simulink model "Excavator_Param_BOFTOF_Calc"  (R2026a)
settings: Solver=ode45  AbsTol=1e-3  EnableMultiTasking=on
PostLoadFcn:
  | if(~exist('bucketForceAngleBOF','var'))
  |    disp('Defining default force angles');
  |    bucketForceAngleBOF = -11.7417;
  |    bucketForceAngleTOF= -1.4472;
  |    bucketForceAngleGravity = -55.5751;
  | end
undefined symbols (not defined in the file or in its folder): A1, A2, B1, B2, B3, BOFTOF_BoomCylArea, BOFTOF_BucketCylArea, BOFTOF_StickCylArea, C1, C2, C3, C4, D1, D2, excv_data, forceTestMaxActiveCylPr, forceTestMaxReactiveCylPr, X, Y, Z
libraries: Excavator_Parts_Param_Lib x21, nesl_utility x12, sm_lib x11, simulink x3, Arrowhead_Lib x1, fl_lib x1
Description:
  | Copyright 2022-2026 The MathWorks, Inc.
settings Model: Creator=smiller  LastModifiedBy=smiller
settings SimscapeCC: ExplicitSolverDiagnosticOptions=none  SimscapeNominalValues="[{\"value\":\"1\",\"unit\":\"A\"},{\"value\":\"1\",\"unit\":\"bar\"},{\"value\":\"1\",\"unit\":\"cm^2\"},{\"value\":\"1\",\"unit\":\"cm^3/s\"},{\"value\":\"1\",\"unit\":\"kJ/kg\"},{\"value\":\"1\",\"unit\":\"kW\"},{\"value\":\"1\",\"unit\":\"l\"},{\"value\":\"1\",\"unit\":\"N\"},{\"value\":\"1\",\"unit\":\"N*m\"},{\"value\":\"1\",\"unit\":\"V\"}]"  SimscapeLogSimulationStatistics=on
settings ExplorerConfigSet: InternalSimMechanicsExplorerSettings="<ExplorerConfiguration><canonicalview>default</canonicalview><AnimationSetting><BasePlaybackSpeed>1.0</BasePlaybackSpeed><PlaybackSpeedFactor>1.0</PlaybackSpeedFactor></AnimationSetting><TilePanel><TileInfo><Tiles Columns=\"1\" Count=\"1\" Rows=\"1\"><Column Weight=\"1\"/><Row Weight=\"1\"/><Tile Height=\"1\" Width=\"1\" X=\"0\" Y=\"0\"/></Tiles></TileInfo><SceneInfo><SceneViewer><BGColor><R>1</R><G>1</G><B>1</B></BGColor><Camera><DoPerspective>off</DoPerspective><Position><X>6.08519841290746477</X><Y>2.23974465526018696</Y><Z>5.98328318454251473</Z></Position><Center><X>6.08519841290746477</X><Y>2.23974465526018696</Y><Z>1.41634799888379348e-07</Z></Center><Up><X>0</X><Y>1</Y><Z>-0</Z></Up><ViewLimDist>1</ViewLimDist><YLim>4.12210355497723135</YLim><XLim>6.50790764061927973</XLim></Camera></SceneViewer></SceneInfo></TilePanel><MechEditorPanel><Cameras/><GfxPanelCameraMap/><VideoCreator><PlaybackSpeedRatio>1.0</PlaybackSpeedRatio><FrameRate>30</FrameRate><VideoFormat>Motion JPEG AVI</VideoFormat><FrameSize>auto</FrameSize></VideoCreator></MechEditorPanel></ExplorerConfiguration>"

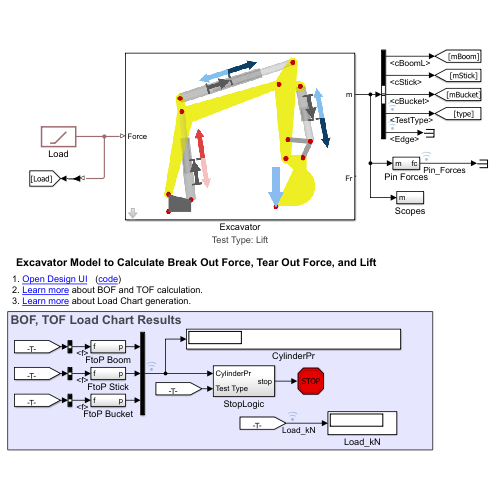
[thumbnail: Simulink's stored preview of the top-level diagram]
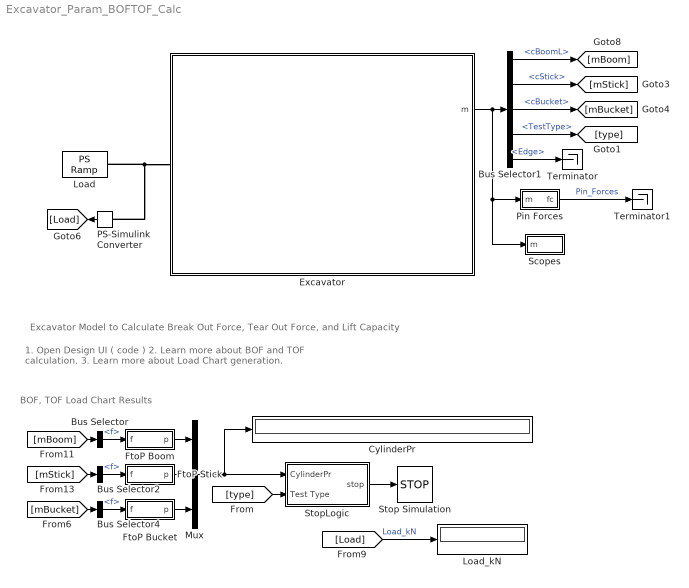
== system Excavator_Param_BOFTOF_Calc ==
  note: BOF, TOF Load Chart Results
  note: Excavator Model to Calculate Break Out Force, Tear Out Force, and Lift Capacity
  note: 1. Open Design UI ( code )
      | 2. Learn more about BOF and TOF calculation.
      | 3. Learn more about Load Chart generation.
  Bus Selector : BusSelector  OutputSignals=f
  Bus Selector1 : BusSelector  OutputSignals=cBoomL,cStick,cBucket,TestType,Edge
  Bus Selector2 : BusSelector  OutputSignals=f
  Bus Selector4 : BusSelector  OutputSignals=f
  CylinderPr : Display
  Excavator : Subsystem  mask{test_type=Lift}
      mask prompts: test_type "Test Type"
      mask init:
      | set_param([gcb '/Apply Force'],'test_type',get_param(gcb,'test_type'));
      | switch(test_type)
      |     case 1
      |         set_param([gcb '/Test Type'],'Value','1');
      |         set_param([gcb '/Mechanism Configuration'],'UniformGravity','None');
      |     case 2
      |         set_param([gcb '/Test Type'],'Value','2');
      |         set_param([gcb '/Mechanism Configuration'],'UniformGravity','None');
      |     case 3
      |         set_param([gcb '/Test Type'],'Value','3');
      |         set_param([gcb '/Mechanism Configuration'],'UniformGravity','Constant');
      | 
      | end
      settings: AttributesFormatString=Test Type: %<test_type>
      mask TypeOptions test_type: BOF | TOF | Lift
      mask Display:
      | switch(get_param(gcb,'test_type'))
      |     case 'BOF'
      |         image('Excavator_Param_Full_CalcForce_BOF_IMAGE.png');
      |     case 'TOF'
      |         image('Excavator_Param_Full_CalcForce_TOF_IMAGE.png');
      |     case 'Lift'
      |         image('Excavator_Param_Full_CalcForce_LoadChart_IMAGE.png');
      | end
  FtoP Boom : Subsystem
  FtoP Bucket : Subsystem
  FtoP Stick : Subsystem
  Load : fl_lib/Physical Signals/Sources/PS Ramp  slope=100 kN/s  start_time=0 s  initial_output=0 kN  ZeroCross=true
  Load_kN : Display
  Mux : Mux  Inputs=3
  PS-Simulink Converter : nesl_utility/PS-Simulink Converter  PhysicalDomain=network_engine_domain  SubClassName=ps_output  LeftPortType=input  RightPortType=output  PseudoPeriodic=off  Frequencies=[]  VectorFormat=inherit  Unit=kN  AffineConversion=off
  Pin Forces : Subsystem
  Scopes : Subsystem
  Stop Simulation : Stop
  StopLogic : Subsystem
  Terminator : Terminator
  Terminator1 : Terminator
  wires:
  PS-Simulink Converter/1 -> [Load]
  Bus Selector1/3 -> [mBucket]  "<cBucket>"
  Excavator/1(m) -> Scopes/1(m), Pin Forces/1(m), Bus Selector1/1
  Bus Selector1/2 -> [mStick]  "<cStick>"
  Bus Selector1/1 -> [mBoom]  "<cBoomL>"
  [mStick] -> Bus Selector2/1
  [mBoom] -> Bus Selector/1
  Bus Selector2/1 -> FtoP Stick/1(f)  "<f>"
  Bus Selector4/1 -> FtoP Bucket/1(f)  "<f>"
  Bus Selector/1 -> FtoP Boom/1(f)  "<f>"
  StopLogic/1(stop) -> Stop Simulation/1
  [Load] -> Load_kN/1  "Load_kN"
  [mBucket] -> Bus Selector4/1
  FtoP Stick/1(p) -> Mux/2
  Mux/1 -> CylinderPr/1, StopLogic/1(CylinderPr)
  FtoP Bucket/1(p) -> Mux/3
  FtoP Boom/1(p) -> Mux/1
  Bus Selector1/4 -> [type]  "<TestType>"
  [type] -> StopLogic/2(Test Type)
  Bus Selector1/5 -> Terminator/1  "<Edge>"
  Pin Forces/1(fc) -> Terminator1/1  "Pin_Forces"
  connections:
  PS-Simulink Converter/LConn1 -- Excavator/LConn1 -- Load/RConn1

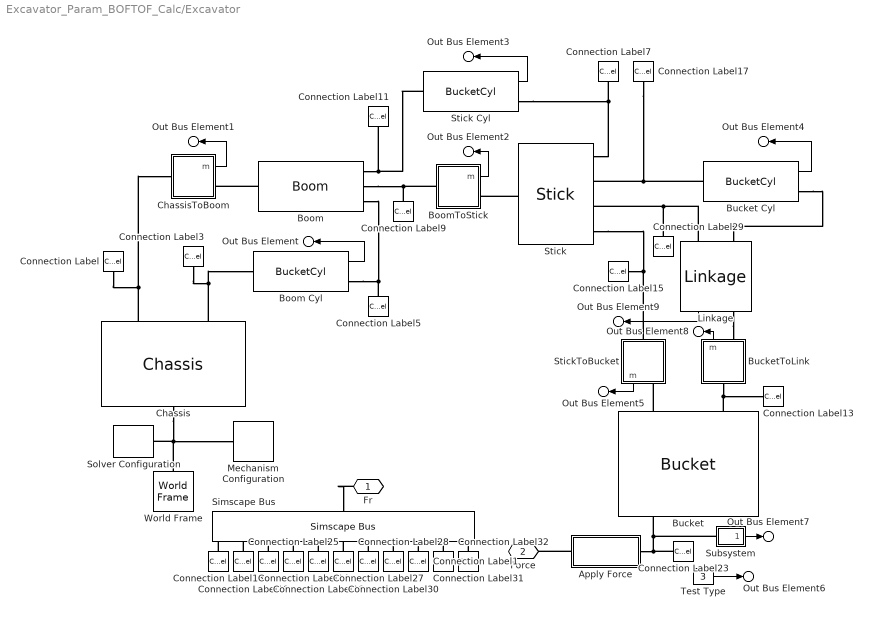
== system Excavator_Param_BOFTOF_Calc/Excavator ==
  Apply Force : Subsystem  mask{test_type=Lift, bof_force_angle=bucketForceAngleBOF, tof_force_angle=bucketForceAngleTOF, lift_force_angle=bucketForceAngleGravity}
      mask prompts: test_type "Test Type"; bof_force_angle "Force Angle, BOF (deg)"; tof_force_angle "Force Angle, TOF (deg)"; lift_force_angle "Force Angle, Lift (deg)"
      mask init:
      | switch(test_type)
      |     case 1
      |         angleCutEdge2BucketForce = bof_force_angle;
      |     case 2
      |         angleCutEdge2BucketForce = tof_force_angle;
      |     case 3
      |         angleCutEdge2BucketForce = lift_force_angle;
      | end
      settings: AttributesFormatString=Test Type: %<test_type>
      mask TypeOptions test_type: BOF | TOF | Lift
  Boom : Excavator_Parts_Param_Lib/Boom  part_thk=excv_data.arm.thk*1.05  part_clr=excv_data.arm.clr  opc=excv_data.arm.opc  pin_len=excv_data.pin.len  pin_rad=excv_data.pin.rad  pin_clr=excv_data.pin.clr  pin_opc=excv_data.pin.opc  Boom=ExcvLocal.Boom  part_mass=LoadChart_BoomMass
  Boom Cyl : Excavator_Parts_Param_Lib/BucketCyl  initPos=initBoomPistonPos  max_force=excv_data.cyl_force.max_force  max_length=excv_data.cyl_force.max_length  arrow_depth=excv_data.cyl_force.depth  line_width=excv_data.cyl_force.line_width  tip_a=90  tip_l=excv_data.cyl_force.tip_length  arrow_clr=excv_data.cyl_force.clr  arrow_opc=excv_data.cyl_force.opc  cyl_len=excv_data.boomcyl.len  cyl_rad=excv_data.cyl.rad  cyl_clr=excv_data.cyl.clr  cyl_opc=excv_data.cyl.opc  pist_len=excv_data.boompist.len  pist_rad=excv_data.pist.rad  pist_clr=excv_data.pist.clr  pist_opc=excv_data.pist.opc
  BoomToStick : Subsystem
      mask Display: image('Excavator_Revolute_IMAGE.png')
  Bucket : Excavator_Parts_Param_Lib/Bucket  part_thk=excv_data.bucket.thk  part_clr=excv_data.bucket.clr  opc=excv_data.arm.opc  pin_len=excv_data.pin.len  pin_rad=excv_data.pin.rad  pin_clr=excv_data.pin.clr  pin_opc=excv_data.pin.opc  Bucket=ExcvLocal.Bucket  part_mass=LoadChart_BucketMass
  Bucket Cyl : Excavator_Parts_Param_Lib/BucketCyl  initPos=initBucketPistonPos  max_force=excv_data.cyl_force.max_force  max_length=excv_data.cyl_force.max_length  arrow_depth=excv_data.cyl_force.depth  line_width=excv_data.cyl_force.line_width  tip_a=90  tip_l=excv_data.cyl_force.tip_length  arrow_clr=excv_data.cyl_force.clr  arrow_opc=excv_data.cyl_force.opc  cyl_len=excv_data.bucketcyl.len  cyl_rad=excv_data.cyl.rad  cyl_clr=excv_data.cyl.clr  cyl_opc=excv_data.cyl.opc  pist_len=excv_data.bucketpist.len  pist_rad=excv_data.pist.rad  pist_clr=excv_data.pist.clr  pist_opc=excv_data.pist.opc
  BucketToLink : Subsystem
      mask Display: image('Excavator_Revolute_IMAGE.png')
  Chassis : Excavator_Parts_Param_Lib/Chassis  Chassis=ExcvLocal.Chassis  opc=excv_data.arm.opc  part_thk=excv_data.chassis.thk  part_clr=excv_data.chassis.clr  pin_clr=excv_data.pin.clr  pin_rad=excv_data.pin.rad  pin_len=excv_data.pin.len  pin_opc=excv_data.pin.opc
  ChassisToBoom : Subsystem
      mask Display: image('Excavator_Revolute_IMAGE.png')
  Connection Label : ConnectionLabel  Label=A1
  Connection Label1 : ConnectionLabel  Label=C4
  Connection Label11 : ConnectionLabel  Label=B2
  Connection Label13 : ConnectionLabel  Label=D1
  Connection Label15 : ConnectionLabel  Label=C4
  Connection Label17 : ConnectionLabel  Label=C2
  Connection Label18 : ConnectionLabel  Label=A1
  Connection Label19 : ConnectionLabel  Label=A2
  Connection Label23 : ConnectionLabel  Label=D2
  Connection Label24 : ConnectionLabel  Label=B1
  Connection Label25 : ConnectionLabel  Label=B2
  Connection Label26 : ConnectionLabel  Label=B3
  Connection Label27 : ConnectionLabel  Label=C1
  Connection Label28 : ConnectionLabel  Label=C2
  Connection Label29 : ConnectionLabel  Label=C3
  Connection Label3 : ConnectionLabel  Label=A2
  Connection Label30 : ConnectionLabel  Label=C3
  Connection Label31 : ConnectionLabel  Label=D1
  Connection Label32 : ConnectionLabel  Label=D2
  Connection Label5 : ConnectionLabel  Label=B1
  Connection Label7 : ConnectionLabel  Label=C1
  Connection Label9 : ConnectionLabel  Label=B3
  Linkage : Excavator_Parts_Param_Lib/Linkage  Linkage=ExcvLocal.Linkage  link_clr=excv_data.link.clr  link_thk=excv_data.link.thk  opc=excv_data.link.opc  pin_clr=excv_data.pin.clr  pin_rad=excv_data.pin.rad  pin_len=excv_data.pin.len  pin_opc=excv_data.pin.opc
  Mechanism Configuration : sm_lib/Utilities/Mechanism Configuration  UniformGravity=Constant  GravityVector=[0 -9.80665 0]  GravityVectorUnits=m/s^2  LinearizationDelta=0.001  JointModeTransitionNonlinearIterations=2
      settings: AttributesFormatString=Gravity: %<UniformGravity>
  Simscape Bus : SimscapeBus  HierarchyStrings=A1;A2;B1;B2;B3;C1;C2;C3;C4;D1;D2
  Solver Configuration : nesl_utility/Solver Configuration  PhysicalDomain=network_engine_domain  SubClassName=solver  LeftPortType=input  RightPortType=generic  Tones=[]  Harmonics=[]  SimulateNoise=off  Profile=off  UseLocalSampling=off  EnableSwitchedLinearOptims=on  FrequencyDomain=off  UseCCode=off  RelTol=0.001  AbsTol=1e-06  MinStep=1e-09  ToWorkspace=off  RevertToSquareIcSolve=off  NumHomotopyIterations=100  PhasorMode=off  PhasorModeNumHarmonics=1  ConsistencySolver=NEWTON_FTOL  CanonicalOrdering=UNORDERED  OptimizeIntermediates=UNOPTIMIZED  IndexReductionMethod=DerivativeReplacement  DoDC=off  ResidualTolerance=1e-09  ConsistencyTolSource=GLOBAL  ConsistencyAbsTol=0.001  ConsistencyRelTol=0.001  ConsistencyTolFactor=0.001  UseLocalSolver=off  LocalSolverChoice=NE_BACKWARD_EULER_ADVANCER  ResolveIndetEquations=on  FunctionEvalNumThread=1  LocalSolverSampleTime=0.001  DoFixedCost=off  MaxNonlinIter=3  MaxModeIter=2  ComputeImpulses=off  ImpulseIterations=2  LinearAlgebra=Sparse  LinearAlgebraNumThread=0  EquationFormulation=NE_TIME_EF  DelaysMemoryBudget=1024  AutomaticFiltering=on  FilteringTimeConstant=0.001  PartitionStorageMethod=AS_NEEDED  PartitionMemoryBudget=1024  PartitionMethod=FAST  MultibodyUseLocalSolver=off  MultibodyLocalSolverChoice=ODE1  MultibodyLocalSolverSampleTime=0.001
  Stick : Excavator_Parts_Param_Lib/Stick  part_thk=excv_data.arm.thk  part_clr=excv_data.arm.clr*0.9  opc=excv_data.arm.opc  pin_len=excv_data.pin.len  pin_rad=excv_data.pin.rad  pin_opc=excv_data.pin.opc  pin_clr=excv_data.pin.clr  Stick=ExcvLocal.Stick  part_mass=LoadChart_StickMass
  Stick Cyl : Excavator_Parts_Param_Lib/BucketCyl  initPos=initStickPistonPos  max_force=excv_data.cyl_force.max_force  max_length=excv_data.cyl_force.max_length  arrow_depth=excv_data.cyl_force.depth  line_width=excv_data.cyl_force.line_width  tip_a=90  tip_l=excv_data.cyl_force.tip_length  arrow_clr=excv_data.cyl_force.clr  arrow_opc=excv_data.cyl_force.opc  cyl_len=excv_data.stickcyl.len  cyl_rad=excv_data.cyl.rad  cyl_clr=excv_data.cyl.clr  cyl_opc=excv_data.cyl.opc  pist_len=excv_data.stickpist.len  pist_rad=excv_data.pist.rad  pist_clr=excv_data.pist.clr  pist_opc=excv_data.pist.opc
  StickToBucket : Subsystem
      mask Display: image('Excavator_Revolute_IMAGE.png')
  Subsystem : Subsystem
  Test Type : Constant  Value=3
  World Frame : sm_lib/Frames and Transforms/World Frame
  Fr : PMIOPort  Side=Right
  Force : PMIOPort  Port=2  Side=Left
  Out Bus Element : Outport  PortName=m  Element=cBoomL
  Out Bus Element3 : Outport  PortName=m  Element=cStick
  Out Bus Element4 : Outport  PortName=m  Element=cBucket
  Out Bus Element1 : Outport  PortName=m  Element=jC2B
  Out Bus Element2 : Outport  PortName=m  Element=jB2S
  Out Bus Element5 : Outport  PortName=m  Element=jS2B
  Out Bus Element6 : Outport  PortName=m  Element=TestType
  Out Bus Element7 : Outport  PortName=m  Element=Edge
  Out Bus Element8 : Outport  PortName=m  Element=jB2L
  Out Bus Element9 : Outport  PortName=m  Element=Linkage
  wires:
  Boom Cyl/1 -> Out Bus Element/1
  Stick Cyl/1 -> Out Bus Element3/1
  Bucket Cyl/1 -> Out Bus Element4/1
  ChassisToBoom/1(m) -> Out Bus Element1/1
  BoomToStick/1(m) -> Out Bus Element2/1
  StickToBucket/1(m) -> Out Bus Element5/1
  Test Type/1 -> Out Bus Element6/1
  Subsystem/1(xy) -> Out Bus Element7/1
  BucketToLink/1(m) -> Out Bus Element8/1
  Linkage/1 -> Out Bus Element9/1
  connections:
  Connection Label24/LConn1 -- Simscape Bus/LConn3
  Connection Label32/LConn1 -- Simscape Bus/LConn11
  Connection Label/LConn1 -- Chassis/RConn1 -- ChassisToBoom/LConn1
  Connection Label29/LConn1 -- Linkage/LConn1 -- Stick/RConn3
  Stick/RConn1 -- Stick Cyl/RConn1 -- Connection Label7/LConn1
  Boom/RConn1 -- Stick Cyl/LConn1 -- Connection Label11/LConn1
  Bucket/LConn1 -- StickToBucket/RConn1
  Connection Label18/LConn1 -- Simscape Bus/LConn1
  Connection Label1/LConn1 -- Simscape Bus/LConn9
  Connection Label5/LConn1 -- Boom Cyl/RConn1 -- Boom/RConn3
  World Frame/RConn1 -- Chassis/LConn1 -- Mechanism Configuration/RConn1 -- Solver Configuration/RConn1
  Connection Label31/LConn1 -- Simscape Bus/LConn10
  Bucket/LConn2 -- Connection Label13/LConn1 -- BucketToLink/LConn1
  Connection Label26/LConn1 -- Simscape Bus/LConn5
  Connection Label28/LConn1 -- Simscape Bus/LConn7
  Connection Label19/LConn1 -- Simscape Bus/LConn2
  Connection Label27/LConn1 -- Simscape Bus/LConn6
  Connection Label25/LConn1 -- Simscape Bus/LConn4
  Connection Label30/LConn1 -- Simscape Bus/LConn8
  Connection Label17/LConn1 -- Bucket Cyl/LConn1 -- Stick/RConn2
  Fr/RConn1 -- Simscape Bus/RConn1
  Connection Label3/LConn1 -- Boom Cyl/LConn1 -- Chassis/RConn2
  Boom/LConn1 -- ChassisToBoom/RConn1
  Connection Label9/LConn1 -- BoomToStick/LConn1 -- Boom/RConn2
  Stick/LConn1 -- BoomToStick/RConn1
  StickToBucket/LConn1 -- Connection Label15/LConn1 -- Stick/RConn4
  Apply Force/LConn1 -- Force/RConn1
  Apply Force/RConn1 -- Connection Label23/LConn1 -- Bucket/RConn1 -- Subsystem/LConn1
  Bucket Cyl/RConn1 -- Linkage/LConn2
  Linkage/RConn1 -- BucketToLink/RConn1

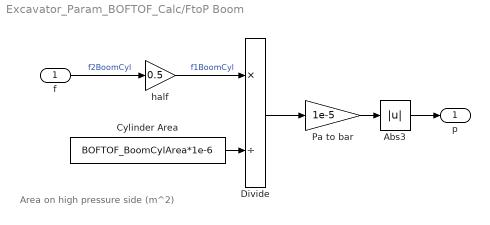
== system Excavator_Param_BOFTOF_Calc/FtoP Boom ==
  note: Area on high pressure side (m^2)
  f : Inport
  Abs3 : Abs  SaturateOnIntegerOverflow=off
  Cylinder Area : Constant  Value=BOFTOF_BoomCylArea*1e-6
  Divide : Product  Inputs=*/
  Pa to bar : Gain  Gain=1e-5
  half : Gain  Gain=0.5
  p : Outport
  wires:
  f/1 -> half/1  "f2BoomCyl"
  Divide/1 -> Pa to bar/1
  half/1 -> Divide/1  "f1BoomCyl"
  Abs3/1 -> p/1
  Pa to bar/1 -> Abs3/1
  Cylinder Area/1 -> Divide/2

== system Excavator_Param_BOFTOF_Calc/FtoP Bucket ==
  note: Area on high pressure side (m^2)
  f : Inport
  Abs1 : Abs  SaturateOnIntegerOverflow=off
  Cylinder Area : Constant  Value=BOFTOF_BucketCylArea*1e-6
  Divide : Product  Inputs=*/
  Pa to bar : Gain  Gain=1e-5
  p : Outport
  wires:
  f/1 -> Divide/1
  Pa to bar/1 -> Abs1/1
  Divide/1 -> Pa to bar/1
  Abs1/1 -> p/1
  Cylinder Area/1 -> Divide/2

== system Excavator_Param_BOFTOF_Calc/FtoP Stick ==
  note: Area on high pressure side (m^2)
  f : Inport
  Abs3 : Abs  SaturateOnIntegerOverflow=off
  Cylinder Area : Constant  Value=BOFTOF_StickCylArea*1e-6
  Divide : Product  Inputs=*/
  Pa to Bar : Gain  Gain=1e-5
  p : Outport
  wires:
  Abs3/1 -> p/1
  Divide/1 -> Pa to Bar/1
  Pa to Bar/1 -> Abs3/1
  f/1 -> Divide/1
  Cylinder Area/1 -> Divide/2

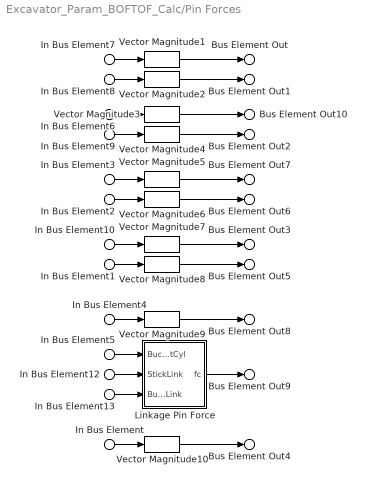
== system Excavator_Param_BOFTOF_Calc/Pin Forces ==
  In Bus Element10 : Inport  PortName=m  Element=cStick.jB.fc
  In Bus Element1 : Inport  PortName=m  Element=cStick.jF.fc
  In Bus Element7 : Inport  PortName=m  Element=jC2B.fc
  In Bus Element8 : Inport  PortName=m  Element=jB2S.fc
  In Bus Element9 : Inport  PortName=m  Element=jS2B.fc
  In Bus Element : Inport  PortName=m  Element=jB2L.fc
  In Bus Element2 : Inport  PortName=m  Element=cBoomL.jB.fc
  In Bus Element3 : Inport  PortName=m  Element=cBoomL.jF.fc
  In Bus Element4 : Inport  PortName=m  Element=cBucket.jB.fc
  In Bus Element5 : Inport  PortName=m  Element=cBucket.jF.fc
  In Bus Element6 : Inport  PortName=m  Element=Linkage.jS2L.fc
  In Bus Element12 : Inport  PortName=m  Element=Linkage.jSL2BC.fc
  In Bus Element13 : Inport  PortName=m  Element=Linkage.jBL2BC.fc
  Linkage Pin Force : Subsystem
  Vector Magnitude{1..10} (10 alike) : Excavator_Parts_Param_Lib/Vector Magnitude  SystemSampleTime=-1  VariantActivationTime=update diagram  EmptyChoice=off  PassThrough=off  PassThroughVariantControl=(default)  EmptyChoiceVariantControl=(default)  AllowFlexibleInterface=on  Latency=0  AutoFrameSizeCalculation=off
  Bus Element Out : Outport  PortName=fc  Element=Boom_To_Chassis
  Bus Element Out1 : Outport  PortName=fc  Element=Boom_To_Stick
  Bus Element Out2 : Outport  PortName=fc  Element=Stick_To_Bucket
  Bus Element Out3 : Outport  PortName=fc  Element=Stick_Cylinder_To_Boom
  Bus Element Out4 : Outport  PortName=fc  Element=Bucket_To_Linkage
  Bus Element Out5 : Outport  PortName=fc  Element=Stick_Cylinder_To_Stick
  Bus Element Out6 : Outport  PortName=fc  Element=Boom_Cylinder_To_Chassis
  Bus Element Out7 : Outport  PortName=fc  Element=Boom_Cylinder_To_Boom
  Bus Element Out8 : Outport  PortName=fc  Element=Bucket_Cylinder_To_Stick
  Bus Element Out9 : Outport  PortName=fc  Element=Bucket_Cylinder_To_Linkage
  Bus Element Out10 : Outport  PortName=fc  Element=Stick_To_Linkage
  wires:
  Vector Magnitude7/1 -> Bus Element Out3/1
  In Bus Element10/1 -> Vector Magnitude7/1
  Vector Magnitude4/1 -> Bus Element Out2/1
  In Bus Element9/1 -> Vector Magnitude4/1
  Vector Magnitude2/1 -> Bus Element Out1/1
  In Bus Element8/1 -> Vector Magnitude2/1
  Vector Magnitude1/1 -> Bus Element Out/1
  In Bus Element7/1 -> Vector Magnitude1/1
  In Bus Element/1 -> Vector Magnitude10/1
  Vector Magnitude10/1 -> Bus Element Out4/1
  Vector Magnitude8/1 -> Bus Element Out5/1
  In Bus Element1/1 -> Vector Magnitude8/1
  In Bus Element2/1 -> Vector Magnitude6/1
  In Bus Element3/1 -> Vector Magnitude5/1
  Vector Magnitude6/1 -> Bus Element Out6/1
  Vector Magnitude5/1 -> Bus Element Out7/1
  In Bus Element4/1 -> Vector Magnitude9/1
  Vector Magnitude9/1 -> Bus Element Out8/1
  In Bus Element6/1 -> Vector Magnitude3/1
  Vector Magnitude3/1 -> Bus Element Out10/1
  In Bus Element5/1 -> Linkage Pin Force/1(BucketCyl)
  In Bus Element12/1 -> Linkage Pin Force/2(StickLink)
  In Bus Element13/1 -> Linkage Pin Force/3(BucketLink)
  Linkage Pin Force/1(fc) -> Bus Element Out9/1

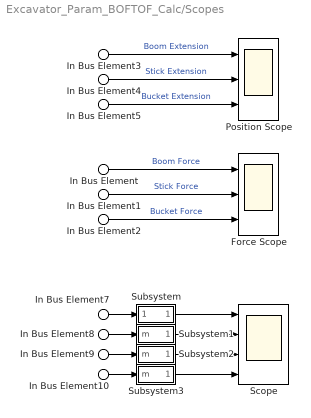
== system Excavator_Param_BOFTOF_Calc/Scopes ==
  In Bus Element : Inport  PortName=m  Element=cBoomL.f
  In Bus Element3 : Inport  PortName=m  Element=cBoomL.pz
  In Bus Element1 : Inport  PortName=m  Element=cStick.f
  In Bus Element4 : Inport  PortName=m  Element=cStick.pz
  In Bus Element10 : Inport  PortName=m  Element=cStick.jB.fc
  In Bus Element2 : Inport  PortName=m  Element=cBucket.f
  In Bus Element5 : Inport  PortName=m  Element=cBucket.pz
  In Bus Element7 : Inport  PortName=m  Element=jC2B.fc
  In Bus Element8 : Inport  PortName=m  Element=jB2S.fc
  In Bus Element9 : Inport  PortName=m  Element=jS2B.fc
  Force Scope : Scope  NumInputPorts=3
      settings: Title=Cylinder Forces  ActiveDisplayYMinimum=-2.01855993393E+6  ActiveDisplayYMaximum=1.89358945982E+6
  Position Scope : Scope  NumInputPorts=3
      settings: ActiveDisplayYMinimum=2036.75361  ActiveDisplayYMaximum=4067.06604
  Scope : Scope  NumInputPorts=4
      settings: ActiveDisplayYMinimum=-225872.14451  ActiveDisplayYMaximum=2.03284930056E+6
  Subsystem : Subsystem
  Subsystem1 : Subsystem
  Subsystem2 : Subsystem
  Subsystem3 : Subsystem
  wires:
  In Bus Element/1 -> Force Scope/1  "Boom Force"
  In Bus Element1/1 -> Force Scope/2  "Stick Force"
  In Bus Element2/1 -> Force Scope/3  "Bucket Force"
  In Bus Element5/1 -> Position Scope/3  "Bucket Extension"
  In Bus Element4/1 -> Position Scope/2  "Stick Extension"
  In Bus Element3/1 -> Position Scope/1  "Boom Extension"
  In Bus Element7/1 -> Subsystem/1(In1)
  Subsystem/1(Out1) -> Scope/1
  In Bus Element8/1 -> Subsystem1/1(m)
  Subsystem1/1(Out1) -> Scope/2
  In Bus Element9/1 -> Subsystem2/1(m)
  Subsystem2/1(Out1) -> Scope/3
  In Bus Element10/1 -> Subsystem3/1(m)
  Subsystem3/1(Out1) -> Scope/4

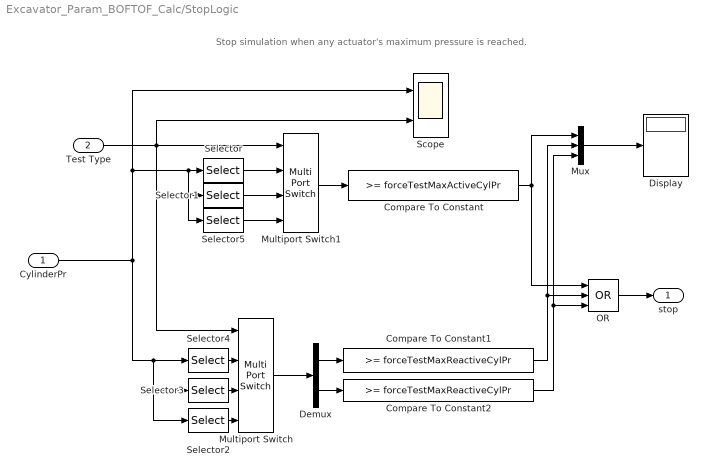
== system Excavator_Param_BOFTOF_Calc/StopLogic ==
  note: Stop simulation when any actuator's maximum pressure is reached.
  CylinderPr : Inport
  Test Type : Inport  Port=2
  Compare To Constant : simulink/Logic and Bit Operations/Compare To Constant  relop=>=  const=forceTestMaxActiveCylPr  OutDataTypeStr=boolean
  Compare To Constant1 : simulink/Logic and Bit Operations/Compare To Constant  relop=>=  const=forceTestMaxReactiveCylPr  OutDataTypeStr=boolean
  Compare To Constant2 : simulink/Logic and Bit Operations/Compare To Constant  relop=>=  const=forceTestMaxReactiveCylPr  OutDataTypeStr=boolean
  Demux : Demux  Outputs=2
  Display : Display
  Multiport Switch : MultiPortSwitch  SaturateOnIntegerOverflow=off  InputSameDT=off
  Multiport Switch1 : MultiPortSwitch  SaturateOnIntegerOverflow=off  InputSameDT=off
  Mux : Mux  Inputs=3
  OR : Logic  Operator=OR  Inputs=3  IconShape=distinctive  AllPortsSameDT=off  OutDataTypeStr=boolean
  Scope : Scope  NumInputPorts=2
      settings: ActiveDisplayYMinimum=-50  ActiveDisplayYMaximum=450
  Selector : Selector  InputPortWidth=3  IndexOptions=Index vector (dialog)  Indices=3  OutputSizes=1
  Selector1 : Selector  InputPortWidth=3  IndexOptions=Index vector (dialog)  Indices=2  OutputSizes=1
  Selector2 : Selector  InputPortWidth=3  IndexOptions=Index vector (dialog)  Indices=[2,3]  OutputSizes=1
  Selector3 : Selector  InputPortWidth=3  IndexOptions=Index vector (dialog)  Indices=[1,3]  OutputSizes=1
  Selector4 : Selector  InputPortWidth=3  IndexOptions=Index vector (dialog)  Indices=[1,2]  OutputSizes=1
  Selector5 : Selector  InputPortWidth=3  IndexOptions=Index vector (dialog)  Indices=1  OutputSizes=1
  stop : Outport
  wires:
  OR/1 -> stop/1
  Compare To Constant2/1 -> OR/3, Mux/3
  Demux/2 -> Compare To Constant2/1
  Demux/1 -> Compare To Constant1/1
  CylinderPr/1 -> Selector4/1, Selector3/1, Selector2/1, Scope/1, Selector5/1, Selector1/1, Selector/1
  Compare To Constant1/1 -> OR/2, Mux/2
  Multiport Switch/1 -> Demux/1
  Compare To Constant/1 -> Mux/1, OR/1
  Multiport Switch1/1 -> Compare To Constant/1
  Selector4/1 -> Multiport Switch/2
  Selector3/1 -> Multiport Switch/3
  Selector1/1 -> Multiport Switch1/3
  Selector/1 -> Multiport Switch1/2
  Mux/1 -> Display/1
  Test Type/1 -> Scope/2, Multiport Switch1/1, Multiport Switch/1
  Selector2/1 -> Multiport Switch/4
  Selector5/1 -> Multiport Switch1/4

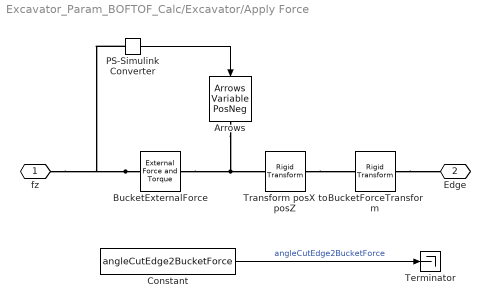
== system Excavator_Param_BOFTOF_Calc/Excavator/Apply Force ==
  Arrows : Arrowhead_Lib/Arrows Variable PosNeg  max_force=4e5  max_length=3  arrow_clr=[0.9019608 0.7058824 0.45490196]  arrow_depth=0.5  line_width=0.2  tip_a=90  tip_l=1  arrow_opc=1
  BucketExternalForce : sm_lib/Forces and Torques/External Force and Torque  EnableForceX=off  EnableForceY=off  EnableForceZ=on  EnableForce=off  ForceResolutionFrame=AttachedFrame  EnableTorqueX=off  EnableTorqueY=off  EnableTorqueZ=off  EnableTorque=off  TorqueResolutionFrame=AttachedFrame
  BucketForceTransform : sm_lib/Frames and Transforms/Rigid Transform  RotationMethod=StandardAxis  FollAlignAxisA=+X  BaseAlignAxisA=+Y  FollAlignAxisB=+Y  BaseAlignAxisB=+Z  RotationStandardAxis=+Z  RotationAngle=angleCutEdge2BucketForce  RotationAngleUnits=deg  RotationArbitraryAxis=[0 0 1]  RotationSequenceAxes=FollowerAxes  RotationSequence=XYX  RotationSequenceAngles=[0 0 0]  RotationSequenceAnglesUnits=deg  RotationMatrix=[1 0 0; 0 1 0; 0 0 1]  Quaternion=[1 0 0 0]  TranslationMethod=None  TranslationCartesianOffset=[0 0 0]  TranslationCartesianOffsetUnits=mm  TranslationStandardAxis=+Z  TranslationStandardOffset=0  TranslationStandardOffsetUnits=mm  TranslationROffset=0  TranslationROffsetUnits=m  TranslationThetaOffset=0  TranslationThetaOffsetUnits=deg  TranslationZOffset=0  TranslationZOffsetUnits=m
  Constant : Constant  Value=angleCutEdge2BucketForce
  PS-Simulink Converter : nesl_utility/PS-Simulink Converter  PhysicalDomain=network_engine_domain  SubClassName=ps_output  LeftPortType=input  RightPortType=output  PseudoPeriodic=off  Frequencies=[]  VectorFormat=inherit  Unit=inherit  AffineConversion=off
  Terminator : Terminator
  Transform posX to posZ : sm_lib/Frames and Transforms/Rigid Transform  RotationMethod=StandardAxis  FollAlignAxisA=+X  BaseAlignAxisA=+Y  FollAlignAxisB=+Y  BaseAlignAxisB=+Z  RotationStandardAxis=+Y  RotationAngle=90  RotationAngleUnits=deg  RotationArbitraryAxis=[0 0 1]  RotationSequenceAxes=FollowerAxes  RotationSequence=XYX  RotationSequenceAngles=[0 0 0]  RotationSequenceAnglesUnits=deg  RotationMatrix=[1 0 0; 0 1 0; 0 0 1]  Quaternion=[1 0 0 0]  TranslationMethod=None  TranslationCartesianOffset=[0 0 0]  TranslationCartesianOffsetUnits=m  TranslationStandardAxis=+Z  TranslationStandardOffset=0  TranslationStandardOffsetUnits=m  TranslationROffset=0  TranslationROffsetUnits=m  TranslationThetaOffset=0  TranslationThetaOffsetUnits=deg  TranslationZOffset=0  TranslationZOffsetUnits=m
  fz : PMIOPort  Side=Left
  Edge : PMIOPort  Port=2  Side=Right
  wires:
  PS-Simulink Converter/1 -> Arrows/1
  Constant/1 -> Terminator/1  "angleCutEdge2BucketForce"
  connections:
  BucketExternalForce/RConn1 -- Transform posX to posZ/RConn1 -- Arrows/RConn1
  Transform posX to posZ/LConn1 -- BucketForceTransform/RConn1
  BucketExternalForce/LConn1 -- PS-Simulink Converter/LConn1 -- fz/RConn1
  BucketForceTransform/LConn1 -- Edge/RConn1

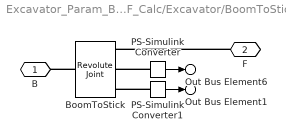
== system Excavator_Param_BOFTOF_Calc/Excavator/BoomToStick ==
  BoomToStick : sm_lib/Joints/Revolute Joint  JointMode=Normal  CompositeWrenchDir=FollowerOnBase  CompositeWrenchFrame=BaseFrame  SenseConstraintForce=on  SenseConstraintTorque=off  SenseTotalForce=off  SenseTotalTorque=off  PositionTargetSpecify=on  PositionTargetPriority=High  PositionTargetValue=initBoomToStickRevPos  PositionTargetValueUnits=deg  VelocityTargetSpecify=off  VelocityTargetPriority=High  VelocityTargetValue=0  VelocityTargetValueUnits=deg/s  EquilibriumPosition=0  EquilibriumPositionUnits=deg  SpringStiffness=0  SpringStiffnessUnits=N*m/deg  DampingCoefficient=0  DampingCoefficientUnits=N*m/(deg/s)  LowerLimitSpecify=off  LowerLimitBound=-90  LowerLimitBoundUnits=deg  LowerLimitStiffness=1e4  LowerLimitStiffnessUnits=N*m/deg  LowerLimitDamping=10  LowerLimitDampingUnits=N*m/(deg/s)  LowerLimitTransitionRegionWidth=0.1  LowerLimitTransitionRegionWidthUnits=deg  UpperLimitSpecify=off  UpperLimitBound=90  UpperLimitBoundUnits=deg  UpperLimitStiffness=1e4  UpperLimitStiffnessUnits=N*m/deg  UpperLimitDamping=10  UpperLimitDampingUnits=N*m/(deg/s)  UpperLimitTransitionRegionWidth=0.1  UpperLimitTransitionRegionWidthUnits=deg  TorqueActuationMode=NoTorque  MotionActuationMode=ComputedMotion  SensePosition=on  SenseVelocity=off  SenseAcceleration=off  SenseTorqueForce=off  SenseLowerLimitTorqueForce=off  SenseUpperLimitTorqueForce=off
  PS-Simulink Converter : nesl_utility/PS-Simulink Converter  PhysicalDomain=network_engine_domain  SubClassName=ps_output  LeftPortType=input  RightPortType=output  PseudoPeriodic=off  Frequencies=[]  VectorFormat=inherit  Unit=deg  AffineConversion=off
  PS-Simulink Converter1 : nesl_utility/PS-Simulink Converter  PhysicalDomain=network_engine_domain  SubClassName=ps_output  LeftPortType=input  RightPortType=output  PseudoPeriodic=off  Frequencies=[]  VectorFormat=inherit  Unit=inherit  AffineConversion=off
  B : PMIOPort  Side=Left
  F : PMIOPort  Port=2  Side=Right
  Out Bus Element6 : Outport  PortName=m  Element=q
  Out Bus Element1 : Outport  PortName=m  Element=fc
  wires:
  PS-Simulink Converter/1 -> Out Bus Element6/1
  PS-Simulink Converter1/1 -> Out Bus Element1/1
  connections:
  BoomToStick/LConn1 -- B/RConn1
  PS-Simulink Converter/LConn1 -- BoomToStick/RConn2
  F/RConn1 -- BoomToStick/RConn1
  PS-Simulink Converter1/LConn1 -- BoomToStick/RConn3

== system Excavator_Param_BOFTOF_Calc/Excavator/BucketToLink ==
  BucketToLink : sm_lib/Joints/Revolute Joint  JointMode=Normal  CompositeWrenchDir=FollowerOnBase  CompositeWrenchFrame=BaseFrame  SenseConstraintForce=on  SenseConstraintTorque=off  SenseTotalForce=off  SenseTotalTorque=off  PositionTargetSpecify=off  PositionTargetPriority=Low  PositionTargetValue=90  PositionTargetValueUnits=deg  VelocityTargetSpecify=off  VelocityTargetPriority=High  VelocityTargetValue=0  VelocityTargetValueUnits=deg/s  EquilibriumPosition=0  EquilibriumPositionUnits=deg  SpringStiffness=0  SpringStiffnessUnits=N*m/deg  DampingCoefficient=0  DampingCoefficientUnits=N*m/(deg/s)  LowerLimitSpecify=off  LowerLimitBound=-90  LowerLimitBoundUnits=deg  LowerLimitStiffness=1e4  LowerLimitStiffnessUnits=N*m/deg  LowerLimitDamping=10  LowerLimitDampingUnits=N*m/(deg/s)  LowerLimitTransitionRegionWidth=0.1  LowerLimitTransitionRegionWidthUnits=deg  UpperLimitSpecify=off  UpperLimitBound=90  UpperLimitBoundUnits=deg  UpperLimitStiffness=1e4  UpperLimitStiffnessUnits=N*m/deg  UpperLimitDamping=10  UpperLimitDampingUnits=N*m/(deg/s)  UpperLimitTransitionRegionWidth=0.1  UpperLimitTransitionRegionWidthUnits=deg  TorqueActuationMode=NoTorque  MotionActuationMode=ComputedMotion  SensePosition=off  SenseVelocity=off  SenseAcceleration=off  SenseTorqueForce=off  SenseLowerLimitTorqueForce=off  SenseUpperLimitTorqueForce=off
  PS-Simulink Converter1 : nesl_utility/PS-Simulink Converter  PhysicalDomain=network_engine_domain  SubClassName=ps_output  LeftPortType=input  RightPortType=output  PseudoPeriodic=off  Frequencies=[]  VectorFormat=inherit  Unit=inherit  AffineConversion=off
  F : PMIOPort  Side=Right
  B : PMIOPort  Port=2  Side=Left
  Out Bus Element1 : Outport  PortName=m  Element=fc
  wires:
  PS-Simulink Converter1/1 -> Out Bus Element1/1
  connections:
  F/RConn1 -- BucketToLink/RConn1
  BucketToLink/LConn1 -- B/RConn1
  BucketToLink/RConn2 -- PS-Simulink Converter1/LConn1

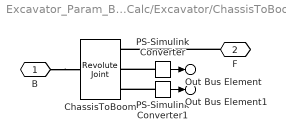
== system Excavator_Param_BOFTOF_Calc/Excavator/ChassisToBoom ==
  ChassisToBoom : sm_lib/Joints/Revolute Joint  JointMode=Normal  CompositeWrenchDir=FollowerOnBase  CompositeWrenchFrame=BaseFrame  SenseConstraintForce=on  SenseConstraintTorque=off  SenseTotalForce=off  SenseTotalTorque=off  PositionTargetSpecify=on  PositionTargetPriority=High  PositionTargetValue=initChassisToBoomRevPos  PositionTargetValueUnits=deg  VelocityTargetSpecify=off  VelocityTargetPriority=High  VelocityTargetValue=0  VelocityTargetValueUnits=deg/s  EquilibriumPosition=0  EquilibriumPositionUnits=deg  SpringStiffness=0  SpringStiffnessUnits=N*m/deg  DampingCoefficient=0  DampingCoefficientUnits=N*m/(deg/s)  LowerLimitSpecify=off  LowerLimitBound=-90  LowerLimitBoundUnits=deg  LowerLimitStiffness=1e4  LowerLimitStiffnessUnits=N*m/deg  LowerLimitDamping=10  LowerLimitDampingUnits=N*m/(deg/s)  LowerLimitTransitionRegionWidth=0.1  LowerLimitTransitionRegionWidthUnits=deg  UpperLimitSpecify=off  UpperLimitBound=90  UpperLimitBoundUnits=deg  UpperLimitStiffness=1e4  UpperLimitStiffnessUnits=N*m/deg  UpperLimitDamping=10  UpperLimitDampingUnits=N*m/(deg/s)  UpperLimitTransitionRegionWidth=0.1  UpperLimitTransitionRegionWidthUnits=deg  TorqueActuationMode=NoTorque  MotionActuationMode=ComputedMotion  SensePosition=on  SenseVelocity=off  SenseAcceleration=off  SenseTorqueForce=off  SenseLowerLimitTorqueForce=off  SenseUpperLimitTorqueForce=off
  PS-Simulink Converter : nesl_utility/PS-Simulink Converter  PhysicalDomain=network_engine_domain  SubClassName=ps_output  LeftPortType=input  RightPortType=output  PseudoPeriodic=off  Frequencies=[]  VectorFormat=inherit  Unit=deg  AffineConversion=off
  PS-Simulink Converter1 : nesl_utility/PS-Simulink Converter  PhysicalDomain=network_engine_domain  SubClassName=ps_output  LeftPortType=input  RightPortType=output  PseudoPeriodic=off  Frequencies=[]  VectorFormat=inherit  Unit=inherit  AffineConversion=off
  B : PMIOPort  Side=Left
  F : PMIOPort  Port=2  Side=Right
  Out Bus Element : Outport  PortName=m  Element=q
  Out Bus Element1 : Outport  PortName=m  Element=fc
  wires:
  PS-Simulink Converter/1 -> Out Bus Element/1
  PS-Simulink Converter1/1 -> Out Bus Element1/1
  connections:
  PS-Simulink Converter/LConn1 -- ChassisToBoom/RConn2
  B/RConn1 -- ChassisToBoom/LConn1
  F/RConn1 -- ChassisToBoom/RConn1
  PS-Simulink Converter1/LConn1 -- ChassisToBoom/RConn3

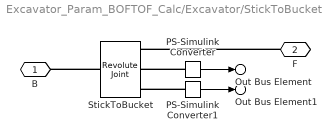
== system Excavator_Param_BOFTOF_Calc/Excavator/StickToBucket ==
  PS-Simulink Converter : nesl_utility/PS-Simulink Converter  PhysicalDomain=network_engine_domain  SubClassName=ps_output  LeftPortType=input  RightPortType=output  PseudoPeriodic=off  Frequencies=[]  VectorFormat=inherit  Unit=deg  AffineConversion=off
  PS-Simulink Converter1 : nesl_utility/PS-Simulink Converter  PhysicalDomain=network_engine_domain  SubClassName=ps_output  LeftPortType=input  RightPortType=output  PseudoPeriodic=off  Frequencies=[]  VectorFormat=inherit  Unit=inherit  AffineConversion=off
  StickToBucket : sm_lib/Joints/Revolute Joint  JointMode=Normal  CompositeWrenchDir=FollowerOnBase  CompositeWrenchFrame=BaseFrame  SenseConstraintForce=on  SenseConstraintTorque=off  SenseTotalForce=off  SenseTotalTorque=off  PositionTargetSpecify=on  PositionTargetPriority=High  PositionTargetValue=initStickToBucketRevPos  PositionTargetValueUnits=deg  VelocityTargetSpecify=off  VelocityTargetPriority=High  VelocityTargetValue=0  VelocityTargetValueUnits=deg/s  EquilibriumPosition=0  EquilibriumPositionUnits=deg  SpringStiffness=0  SpringStiffnessUnits=N*m/deg  DampingCoefficient=0  DampingCoefficientUnits=N*m/(deg/s)  LowerLimitSpecify=off  LowerLimitBound=-90  LowerLimitBoundUnits=deg  LowerLimitStiffness=1e4  LowerLimitStiffnessUnits=N*m/deg  LowerLimitDamping=10  LowerLimitDampingUnits=N*m/(deg/s)  LowerLimitTransitionRegionWidth=0.1  LowerLimitTransitionRegionWidthUnits=deg  UpperLimitSpecify=off  UpperLimitBound=90  UpperLimitBoundUnits=deg  UpperLimitStiffness=1e4  UpperLimitStiffnessUnits=N*m/deg  UpperLimitDamping=10  UpperLimitDampingUnits=N*m/(deg/s)  UpperLimitTransitionRegionWidth=0.1  UpperLimitTransitionRegionWidthUnits=deg  TorqueActuationMode=NoTorque  MotionActuationMode=ComputedMotion  SensePosition=on  SenseVelocity=off  SenseAcceleration=off  SenseTorqueForce=off  SenseLowerLimitTorqueForce=off  SenseUpperLimitTorqueForce=off
  B : PMIOPort  Side=Left
  F : PMIOPort  Port=2  Side=Right
  Out Bus Element : Outport  PortName=m  Element=q
  Out Bus Element1 : Outport  PortName=m  Element=fc
  wires:
  PS-Simulink Converter/1 -> Out Bus Element/1
  PS-Simulink Converter1/1 -> Out Bus Element1/1
  connections:
  F/RConn1 -- StickToBucket/RConn1
  StickToBucket/LConn1 -- B/RConn1
  PS-Simulink Converter/LConn1 -- StickToBucket/RConn2
  PS-Simulink Converter1/LConn1 -- StickToBucket/RConn3

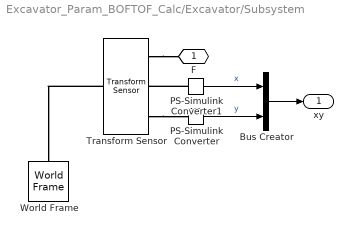
== system Excavator_Param_BOFTOF_Calc/Excavator/Subsystem ==
  Bus Creator : BusCreator  Inputs=2
  PS-Simulink Converter : nesl_utility/PS-Simulink Converter  PhysicalDomain=network_engine_domain  SubClassName=ps_output  LeftPortType=input  RightPortType=output  PseudoPeriodic=off  Frequencies=[]  VectorFormat=inherit  Unit=inherit  AffineConversion=off
  PS-Simulink Converter1 : nesl_utility/PS-Simulink Converter  PhysicalDomain=network_engine_domain  SubClassName=ps_output  LeftPortType=input  RightPortType=output  PseudoPeriodic=off  Frequencies=[]  VectorFormat=inherit  Unit=inherit  AffineConversion=off
  Transform Sensor : sm_lib/Frames and Transforms/Transform Sensor  MeasurementFrame=World  RotationSequence=XYX  SenseAngle=off  SenseAxis=off  SenseQ=off  SenseR=off  SenseRotationSequence=off  SenseOmegaX=off  SenseOmegaY=off  SenseOmegaZ=off  SenseOmega=off  SenseQDot=off  SenseRDot=off  SenseRotationSequenceDot=off  SenseAlphaX=off  SenseAlphaY=off  SenseAlphaZ=off  SenseAlpha=off  SenseQDDot=off  SenseRDDot=off  SenseX=on  SenseY=on  SenseZ=off  SenseXYZ=off  SenseRad=off  SenseAzim=off  SenseDist=off  SenseInc=off  SenseXDot=off  SenseYDot=off  SenseZDot=off  SenseXYZDot=off  SenseRadDot=off  SenseAzimDot=off  SenseDistDot=off  SenseIncDot=off  SenseXDDot=off  SenseYDDot=off  SenseZDDot=off  SenseXYZDDot=off  SenseRadDDot=off  SenseAzimDDot=off  SenseDistDDot=off  SenseIncDDot=off
  World Frame : sm_lib/Frames and Transforms/World Frame
  F : PMIOPort  Side=Left
  xy : Outport
  wires:
  PS-Simulink Converter/1 -> Bus Creator/2  "y"
  PS-Simulink Converter1/1 -> Bus Creator/1  "x"
  Bus Creator/1 -> xy/1
  connections:
  Transform Sensor/RConn1 -- F/RConn1
  Transform Sensor/LConn1 -- World Frame/RConn1
  Transform Sensor/RConn3 -- PS-Simulink Converter/LConn1
  PS-Simulink Converter1/LConn1 -- Transform Sensor/RConn2

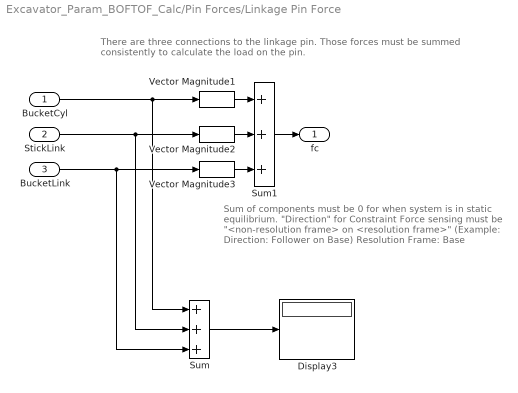
== system Excavator_Param_BOFTOF_Calc/Pin Forces/Linkage Pin Force ==
  note: There are three connections to the linkage pin. Those forces must be summed consistently to calculate the load on the pin.
  note: Sum of components must be 0 for when system
      | is in static equilibrium. "Direction" for
      | Constraint Force sensing must be
      | "<non-resolution frame> on <resolution frame>"
      | (Example: Direction: Follower on Base)
      |                  Resolution Frame: Base
  BucketCyl : Inport
  StickLink : Inport  Port=2
  BucketLink : Inport  Port=3
  Display3 : Display
  Sum : Sum  Inputs=+++
  Sum1 : Sum  Inputs=+++
  Vector Magnitude1 : Excavator_Parts_Param_Lib/Vector Magnitude  SystemSampleTime=-1  VariantActivationTime=update diagram  EmptyChoice=off  PassThrough=off  PassThroughVariantControl=(default)  EmptyChoiceVariantControl=(default)  AllowFlexibleInterface=on  Latency=0  AutoFrameSizeCalculation=off
  Vector Magnitude2 : Excavator_Parts_Param_Lib/Vector Magnitude  SystemSampleTime=-1  VariantActivationTime=update diagram  EmptyChoice=off  PassThrough=off  PassThroughVariantControl=(default)  EmptyChoiceVariantControl=(default)  AllowFlexibleInterface=on  Latency=0  AutoFrameSizeCalculation=off
  Vector Magnitude3 : Excavator_Parts_Param_Lib/Vector Magnitude  SystemSampleTime=-1  VariantActivationTime=update diagram  EmptyChoice=off  PassThrough=off  PassThroughVariantControl=(default)  EmptyChoiceVariantControl=(default)  AllowFlexibleInterface=on  Latency=0  AutoFrameSizeCalculation=off
  fc : Outport
  wires:
  Sum1/1 -> fc/1
  Vector Magnitude2/1 -> Sum1/2
  Vector Magnitude3/1 -> Sum1/3
  Vector Magnitude1/1 -> Sum1/1
  StickLink/1 -> Vector Magnitude2/1, Sum/2
  BucketCyl/1 -> Vector Magnitude1/1, Sum/1
  BucketLink/1 -> Vector Magnitude3/1, Sum/3
  Sum/1 -> Display3/1

== system Excavator_Param_BOFTOF_Calc/Scopes/Subsystem ==
  In1 : Inport
  Dot Product : DotProduct  OutDataTypeStr=Inherit: Inherit via internal rule
  Sqrt : Sqrt
  Out1 : Outport
  wires:
  In1/1 -> Dot Product/1, Dot Product/2
  Dot Product/1 -> Sqrt/1
  Sqrt/1 -> Out1/1

== system Excavator_Param_BOFTOF_Calc/Scopes/Subsystem1 ==
  m : Inport
  Dot Product : DotProduct  OutDataTypeStr=Inherit: Inherit via internal rule
  Sqrt : Sqrt
  Out1 : Outport
  wires:
  Sqrt/1 -> Out1/1
  Dot Product/1 -> Sqrt/1
  m/1 -> Dot Product/2, Dot Product/1

== system Excavator_Param_BOFTOF_Calc/Scopes/Subsystem2 ==
  m : Inport
  Dot Product : DotProduct  OutDataTypeStr=Inherit: Inherit via internal rule
  Sqrt : Sqrt
  Out1 : Outport
  wires:
  m/1 -> Dot Product/1, Dot Product/2
  Dot Product/1 -> Sqrt/1
  Sqrt/1 -> Out1/1

== system Excavator_Param_BOFTOF_Calc/Scopes/Subsystem3 ==
  m : Inport
  Dot Product : DotProduct  OutDataTypeStr=Inherit: Inherit via internal rule
  Sqrt : Sqrt
  Out1 : Outport
  wires:
  Sqrt/1 -> Out1/1
  Dot Product/1 -> Sqrt/1
  m/1 -> Dot Product/2, Dot Product/1
